simulink model "LaneFollowingNMPC"  (R2020a)
settings: Solver=FixedStepAuto  StartTime=0.0  StopTime=Duration  FixedStep=0.1  RelTol=1e-3  EnableMultiTasking=on
PreLoadFcn:
  | LaneFollowingUsingNMPCData
values from neighbouring files (symbols this model uses):
  Cf = 19000    [LaneFollowingUsingNMPCData.m]
  Cr = 33000    [LaneFollowingUsingNMPCData.m]
  Iz = 2875    [LaneFollowingUsingNMPCData.m]
  lf = 1.2    [LaneFollowingUsingNMPCData.m]
  lr = 1.6    [LaneFollowingUsingNMPCData.m]
  m = 1575    [LaneFollowingUsingNMPCData.m]
  rho = LaneFollowingGetCurvature(v_set,t)    [LaneFollowingUsingNMPCData.m]
  tau = 0.2    [LaneFollowingUsingNMPCData.m]
  Ts = u(5)    [LaneFollowingEKFStateFcn.m]    (also in LaneFollowingUsingNMPCData.m = 0.1)
  v0 = 15    [LaneFollowingUsingNMPCData.m]
  v_set = 20    [LaneFollowingUsingNMPCData.m]
libraries: sharedTrackingLibrary x1, forceslib x1
settings Model: NumberOfSteps=3  Creator=The MathWorks, Inc.  LastModifiedBy=j-hho
settings SolverCC: ConcurrentTasks=on  AutoInsertRateTranBlk=on
settings DataIOCC: SaveFormat=StructureWithTime  ReturnWorkspaceOutputs=off
settings OptimizationCC: BlockReduction=off  OptimizeBlockIOStorage=off
settings DebuggingCC: PregeneratedLibrarySubsystemCodeDiagnostic=none  ArithmeticOperatorsInVariantConditions=warning
settings HardwareCC: ProdBitPerPointer=32  ProdBitPerSizeT=32  ProdBitPerPtrDiffT=32  ProdLargestAtomicFloat=None  ProdWordSize=32  ProdLongLongMode=on  ProdHWDeviceType=Generic->32-bit x86 compatible
settings SFSimCC: SimUseLocalCustomCode=off  CustomCodeUndefinedFunction=UseInterfaceOnly
settings RTWCC: Description=Generic Real-Time Target  RTWUseLocalCustomCode=off  RTWCompilerOptimization=on
settings CodeAppCC: StateflowObjectComments=on
settings GRTTargetCC: TargetLangStandard=C89/C90 (ANSI)
settings SimscapeCC: SimscapeNormalizeSystem=off

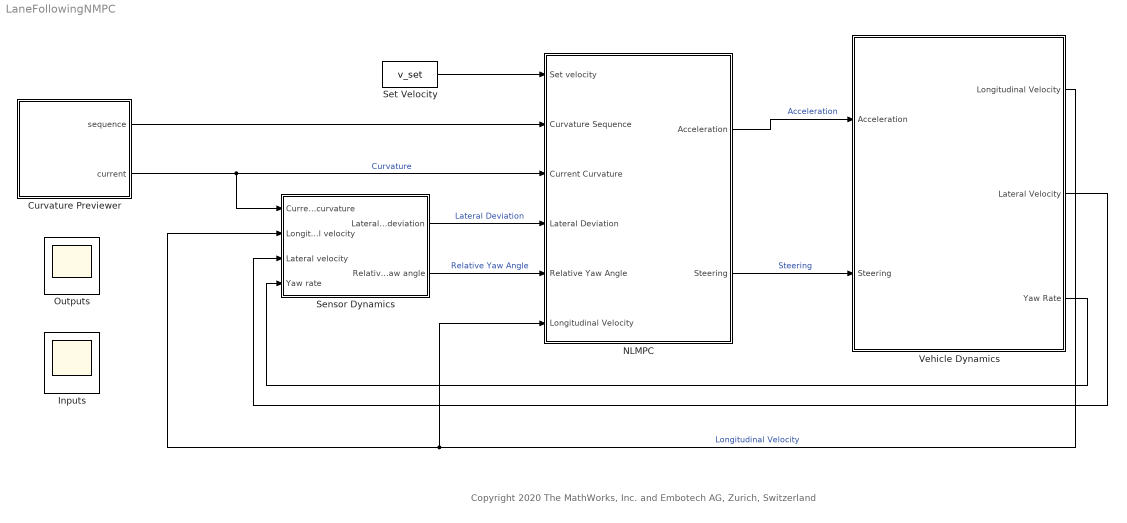
== system LaneFollowingNMPC ==
  note: Copyright 2020 The MathWorks, Inc. and Embotech AG, Zurich, Switzerland
  Curvature Previewer : Subsystem  mask{signal=rho, ts=Ts, steps=10}
      mask prompts: signal "Signal name"; ts "Sampling time"; steps "Number of previewing steps"
      mask init:
      | ts = evalin('base',get_param(gcbh,'ts'));
      | signal = evalin('base',get_param(gcbh,'signal'));
      | steps = evalin('base',get_param(gcbh,'steps'));
      | data = mpc_previewer_maskinit(signal,ts);
      mask Display:
      | fprintf('Future\nsample\nextractor');
      | port_label('output', 1, 'seq')
      | port_label('output', 2, '@t')
  Inputs : Scope
      settings: Floating=on
  NLMPC : Subsystem  VariantControl=controller_type ==1
  Outputs : Scope
      settings: Floating=on
  Sensor Dynamics : Subsystem
  Set Velocity : Constant  Value=v_set
  Vehicle Dynamics : Subsystem
  wires:
  Curvature Previewer/2(current) -> NLMPC/3(Current Curvature), Sensor Dynamics/1(Current curvature)  "Curvature"
  Vehicle Dynamics/2(Lateral Velocity) -> Sensor Dynamics/3(Lateral velocity)
  Vehicle Dynamics/3(Yaw Rate) -> Sensor Dynamics/4(Yaw rate)
  Vehicle Dynamics/1(Longitudinal Velocity) -> NLMPC/6(Longitudinal Velocity), Sensor Dynamics/2(Longitudinal velocity)  "Longitudinal Velocity"
  Curvature Previewer/1(sequence) -> NLMPC/2(Curvature Sequence)
  Sensor Dynamics/1(Lateral deviation) -> NLMPC/4(Lateral Deviation)  "Lateral Deviation"
  Sensor Dynamics/2(Relative yaw angle) -> NLMPC/5(Relative Yaw Angle)  "Relative Yaw Angle"
  Set Velocity/1 -> NLMPC/1(Set velocity)
  NLMPC/1(Acceleration) -> Vehicle Dynamics/1(Acceleration)  "Acceleration"
  NLMPC/2(Steering) -> Vehicle Dynamics/2(Steering)  "Steering"

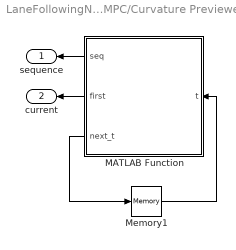
== system LaneFollowingNMPC/Curvature Previewer ==
  MATLAB Function : MATLAB Function  TreatAsAtomicUnit=on
  Memory1 : Memory  InheritSampleTime=on  LinearizeAsDelay=on
  sequence : Outport  VectorParamsAs1DForOutWhenUnconnected=off
  current : Outport  Port=2  VectorParamsAs1DForOutWhenUnconnected=off
  wires:
  MATLAB Function/1(seq) -> sequence/1
  MATLAB Function/2(first) -> current/1
  Memory1/1 -> MATLAB Function/1(t)
  MATLAB Function/3(next_t) -> Memory1/1

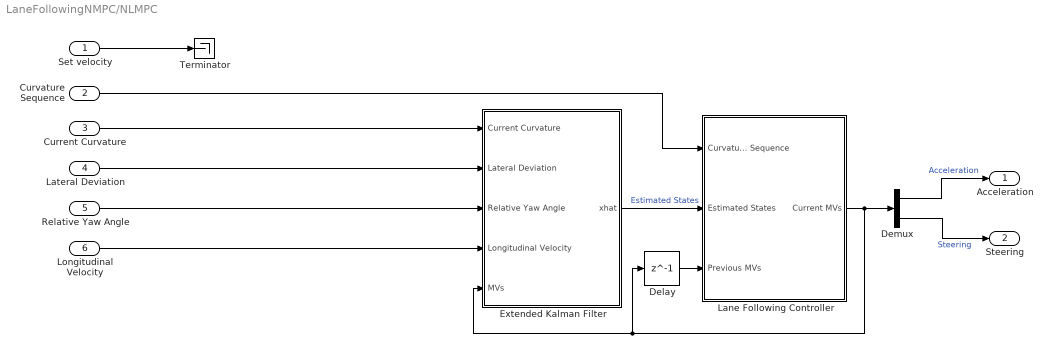
== system LaneFollowingNMPC/NLMPC ==
  Set velocity : Inport
  Curvature Sequence : Inport  Port=2
  Current Curvature : Inport  Port=3
  Lateral Deviation : Inport  Port=4
  Relative Yaw Angle : Inport  Port=5
  Longitudinal Velocity : Inport  Port=6
  Delay : Delay  DelayLength=1  InitialCondition=[0.2 0.3]
  Demux : Demux  Outputs=2
  Extended Kalman Filter : Subsystem
  Lane Following Controller : Subsystem
  Terminator : Terminator
  Acceleration : Outport  VectorParamsAs1DForOutWhenUnconnected=off
  Steering : Outport  Port=2  VectorParamsAs1DForOutWhenUnconnected=off
  wires:
  Extended Kalman Filter/1(xhat) -> Lane Following Controller/2(Estimated States)  "Estimated States"
  Lane Following Controller/1(Current MVs) -> Demux/1, Extended Kalman Filter/5(MVs), Delay/1
  Lateral Deviation/1 -> Extended Kalman Filter/2(Lateral Deviation)
  Curvature Sequence/1 -> Lane Following Controller/1(Curvature Sequence)
  Longitudinal Velocity/1 -> Extended Kalman Filter/4(Longitudinal Velocity)
  Delay/1 -> Lane Following Controller/3(Previous MVs)
  Relative Yaw Angle/1 -> Extended Kalman Filter/3(Relative Yaw Angle)
  Current Curvature/1 -> Extended Kalman Filter/1(Current Curvature)
  Set velocity/1 -> Terminator/1
  Demux/2 -> Steering/1  "Steering"
  Demux/1 -> Acceleration/1  "Acceleration"

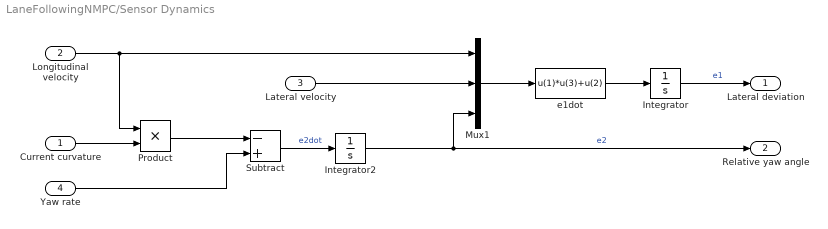
== system LaneFollowingNMPC/Sensor Dynamics ==
  Current curvature : Inport
  Longitudinal velocity : Inport  Port=2
  Lateral velocity : Inport  Port=3
  Yaw rate : Inport  Port=4
  Integrator : Integrator
  Integrator2 : Integrator
  Mux1 : Mux  Inputs=[1 1 1]
  Product : Product
  Subtract : Sum  Inputs=-+
  e1dot : Fcn  Expr=u(1)*u(3)+u(2)
  Lateral deviation : Outport  VectorParamsAs1DForOutWhenUnconnected=off
  Relative yaw angle : Outport  Port=2  VectorParamsAs1DForOutWhenUnconnected=off
  wires:
  Current curvature/1 -> Product/2
  Mux1/1 -> e1dot/1
  e1dot/1 -> Integrator/1
  Longitudinal velocity/1 -> Product/1, Mux1/1
  Lateral velocity/1 -> Mux1/2
  Integrator/1 -> Lateral deviation/1  "e1"
  Product/1 -> Subtract/1
  Yaw rate/1 -> Subtract/2
  Subtract/1 -> Integrator2/1  "e2dot"
  Integrator2/1 -> Mux1/3, Relative yaw angle/1  "e2"

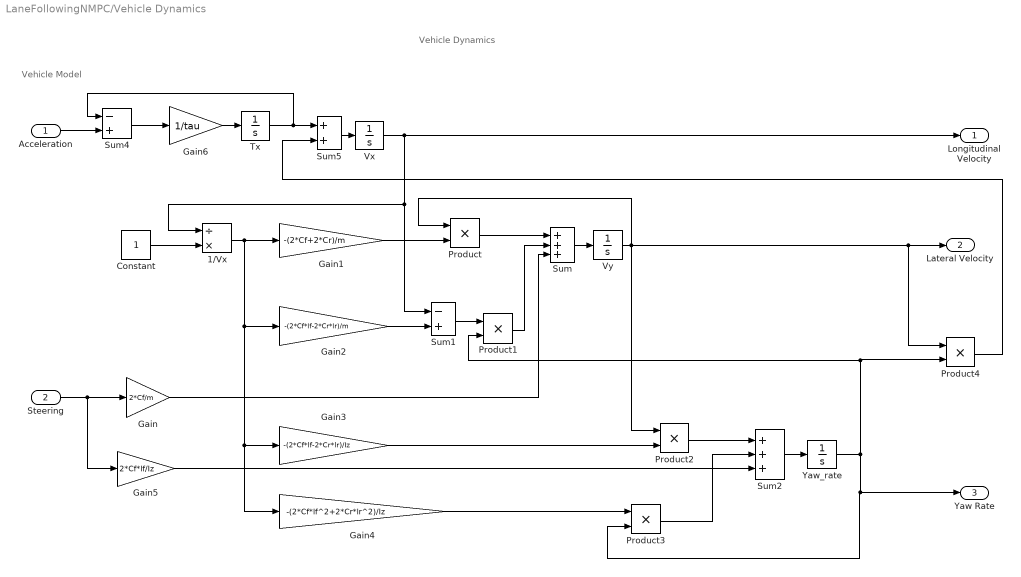
== system LaneFollowingNMPC/Vehicle Dynamics ==
  note: Vehicle Model
  note: Vehicle Dynamics
  Acceleration : Inport
  Steering : Inport  Port=2
  1/Vx : Product  Inputs=/*
  Constant : Constant
  Gain : Gain  Gain=2*Cf/m
  Gain1 : Gain  Gain=-(2*Cf+2*Cr)/m
  Gain2 : Gain  Gain=-(2*Cf*lf-2*Cr*lr)/m
  Gain3 : Gain  Gain=-(2*Cf*lf-2*Cr*lr)/Iz
  Gain4 : Gain  Gain=-(2*Cf*lf^2+2*Cr*lr^2)/Iz
  Gain5 : Gain  Gain=2*Cf*lf/Iz
  Gain6 : Gain  Gain=1/tau
  Product{,1..4} (5 alike) : Product
  Sum : Sum  Inputs=+++
  Sum1 : Sum  Inputs=-+
  Sum2 : Sum  Inputs=+++
  Sum4 : Sum  Inputs=-+
  Sum5 : Sum
  Tx : Integrator
  Vx : Integrator  InitialCondition=v0
  Vy : Integrator
  "Yaw_rate " : Integrator
  Longitudinal Velocity : Outport  VectorParamsAs1DForOutWhenUnconnected=off
  Lateral Velocity : Outport  Port=2  VectorParamsAs1DForOutWhenUnconnected=off
  Yaw Rate : Outport  Port=3  VectorParamsAs1DForOutWhenUnconnected=off
  wires:
  Gain6/1 -> Tx/1
  Sum2/1 -> "Yaw_rate "/1
  Sum5/1 -> Vx/1
  Gain2/1 -> Sum1/2
  Gain4/1 -> Product3/1
  Constant/1 -> 1/Vx/2
  Gain3/1 -> Product2/2
  1/Vx/1 -> Gain4/1, Gain3/1, Gain2/1, Gain1/1
  Product2/1 -> Sum2/1
  Sum4/1 -> Gain6/1
  Acceleration/1 -> Sum4/2
  Tx/1 -> Sum5/1, Sum4/1
  Product3/1 -> Sum2/2
  Gain5/1 -> Sum2/3
  Product4/1 -> Sum5/2
  Sum1/1 -> Product1/1
  "Yaw_rate "/1 -> Yaw Rate/1, Product3/2, Product4/2, Product1/2
  Gain/1 -> Sum/3
  Steering/1 -> Gain/1, Gain5/1
  Gain1/1 -> Product/2
  Product/1 -> Sum/1
  Vy/1 -> Product/1, Lateral Velocity/1, Product4/1, Product2/1
  Sum/1 -> Vy/1
  Vx/1 -> Longitudinal Velocity/1, 1/Vx/1, Sum1/1
  Product1/1 -> Sum/2

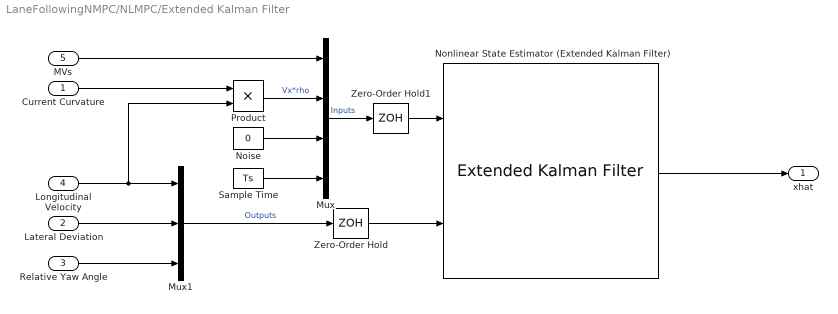
== system LaneFollowingNMPC/NLMPC/Extended Kalman Filter ==
  Current Curvature : Inport
  Lateral Deviation : Inport  Port=2
  Relative Yaw Angle : Inport  Port=3
  Longitudinal Velocity : Inport  Port=4
  MVs : Inport  Port=5
  Mux : Mux
  Mux1 : Mux  Inputs=3
  Noise : Constant  Value=0
  Nonlinear State Estimator (Extended Kalman Filter) : sharedTrackingLibrary/Extended Kalman Filter  StateTransitionFcn=LaneFollowingEKFStateFcn  HasStateTransitionJacobianFcn=off  HasAdditiveProcessNoise=Additive  ProcessNoise=1e-4*eye(7)  HasTimeVaryingProcessNoise=off  HasStateTransitionFcnExtraArgument=1  InitialState=[0 0 v0 0 0 0 0]'  InitialStateCovariance=1e-4*eye(7)  MeasurementFcn1=LaneFollowingEKFMeasFcn  HasMeasurementJacobianFcn1=off  HasMeasurementEnablePort1=off  HasAdditiveMeasurementNoise1=Additive  MeasurementNoise1=1e-4*eye(3)  HasTimeVaryingMeasurementNoise1=off  HasMeasurementFcnExtraArgument1=0  MeasurementFcn2=myMeasurementFcn  HasMeasurementJacobianFcn2=off  HasMeasurementEnablePort2=off  HasAdditiveMeasurementNoise2=Additive  MeasurementNoise2=1  HasTimeVaryingMeasurementNoise2=off  HasMeasurementFcnExtraArgument2=0  MeasurementFcn3=myMeasurementFcn  HasMeasurementJacobianFcn3=off  HasMeasurementEnablePort3=off  HasAdditiveMeasurementNoise3=Additive  MeasurementNoise3=1  HasTimeVaryingMeasurementNoise3=off  HasMeasurementFcnExtraArgument3=0  MeasurementFcn4=myMeasurementFcn  HasMeasurementJacobianFcn4=off  HasMeasurementEnablePort4=off  HasAdditiveMeasurementNoise4=Additive  MeasurementNoise4=1  HasTimeVaryingMeasurementNoise4=off  HasMeasurementFcnExtraArgument4=0  MeasurementFcn5=myMeasurementFcn  HasMeasurementJacobianFcn5=off  HasMeasurementEnablePort5=off  HasAdditiveMeasurementNoise5=Additive  MeasurementNoise5=1  HasTimeVaryingMeasurementNoise5=off  HasMeasurementFcnExtraArgument5=0  EnableMultirate=off  StateTransitionFcnSampleTime=1  MeasurementFcn1SampleTime=1  MeasurementFcn2SampleTime=1  MeasurementFcn3SampleTime=1  MeasurementFcn4SampleTime=1  MeasurementFcn5SampleTime=1  UseCurrentEstimator=on  OutputStateCovariance=off  DataType=double  SampleTime=Ts  NumberOfMeasurements=1
      settings: SourceProductBaseCode=CT,DR,TF,ID,NV,AR,RO,VE
  Product : Product
  Sample Time : Constant  Value=Ts
  Zero-Order Hold : ZeroOrderHold  SampleTime=Ts
  Zero-Order Hold1 : ZeroOrderHold  SampleTime=Ts
  xhat : Outport  VectorParamsAs1DForOutWhenUnconnected=off
  wires:
  Noise/1 -> Mux/3
  Zero-Order Hold/1 -> Nonlinear State Estimator (Extended Kalman Filter)/2
  MVs/1 -> Mux/1
  Sample Time/1 -> Mux/4
  Nonlinear State Estimator (Extended Kalman Filter)/1 -> xhat/1
  Mux1/1 -> Zero-Order Hold/1  "Outputs"
  Lateral Deviation/1 -> Mux1/2
  Longitudinal Velocity/1 -> Mux1/1, Product/2
  Relative Yaw Angle/1 -> Mux1/3
  Current Curvature/1 -> Product/1
  Product/1 -> Mux/2  "Vx*rho"
  Mux/1 -> Zero-Order Hold1/1  "Inputs"
  Zero-Order Hold1/1 -> Nonlinear State Estimator (Extended Kalman Filter)/1

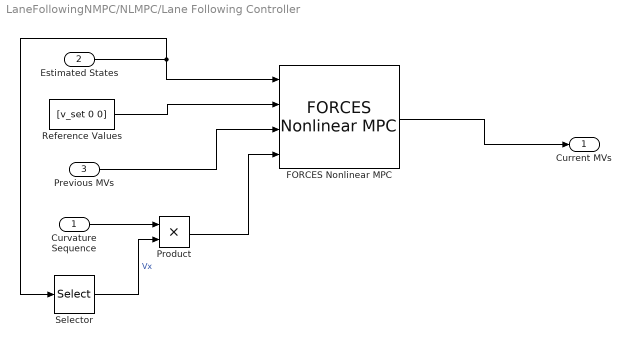
== system LaneFollowingNMPC/NLMPC/Lane Following Controller ==
  Curvature Sequence : Inport
  Estimated States : Inport  Port=2
  Previous MVs : Inport  Port=3
  FORCES Nonlinear MPC : forceslib/FORCES Nonlinear MPC  SCDEnableBlockLinearizationSpecification=on  nlmpcobj=coredata  UseObjectTs=on  md_enabled=on  mvtarget_enabled=off  param_enabled=off  cost_enabled=off  mvseq_enabled=off  stateseq_enabled=off  ovseq_enabled=off  status_enabled=off  ov_min=off  ov_max=off  mv_min=off  mv_max=off  mvrate_min=off  mvrate_max=off  state_min=off  state_max=off  ov_weight=off  mv_weight=off  mvrate_weight=off  ecr_weight=off  nlp_initialize=off
      settings: SourceProductName=FORCES PRO MPC Blocks
  Product : Product
  Reference Values : Constant  Value=[v_set 0 0]  VectorParams1D=off
  Selector : Selector  InputPortWidth=7  IndexOptions=Index vector (dialog)  Indices=[3]  OutputSizes=1
  Current MVs : Outport  VectorParamsAs1DForOutWhenUnconnected=off
  wires:
  Estimated States/1 -> FORCES Nonlinear MPC/1, Selector/1
  Selector/1 -> Product/2  "Vx"
  Curvature Sequence/1 -> Product/1
  Reference Values/1 -> FORCES Nonlinear MPC/2
  Previous MVs/1 -> FORCES Nonlinear MPC/3
  FORCES Nonlinear MPC/1 -> Current MVs/1
  Product/1 -> FORCES Nonlinear MPC/4

== matlab function LaneFollowingNMPC/Curvature Previewer/MATLAB Function ==
  settings: updateMethod=DISCRETE  sampleTime=ts
  data: data parameter; seq output; steps parameter; t input; first output; next_t output
function [seq,first,next_t] = fcn(data,steps,t)
%#codegen
[seq,first,next_t] = mpcblock_preview('md',data,steps,t);
